simulink model "SlidesExampleNew"  (Simulink 7.4)
settings: Solver=FixedStepDiscrete  StartTime=0.0  StopTime=120  FixedStep=0.5  MaxStep=1  RelTol=1e-3
values from neighbouring files (symbols this model uses):
  y0 = -20    [SlidesExampleMfile.m]
undefined symbols (not defined in the file or in its folder): BLOM_FunctionCode, thetak, vk, xk, yk
libraries: BLOM_Lib x10
settings Model: Creator=vichik  LastModifiedBy=Kyle
settings OptimizationCC: InitFltsAndDblsToZero=on
settings DebuggingCC: StrictBusMsg=ErrorLevel1

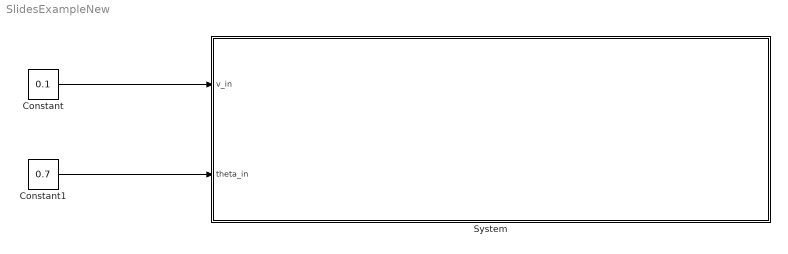
== system SlidesExampleNew ==
  Constant : Constant  Value=0.1
  Constant1 : Constant  Value=0.7
  System : Subsystem
  wires:
  Constant/1 -> System/1(v_in)
  Constant1/1 -> System/2(theta_in)

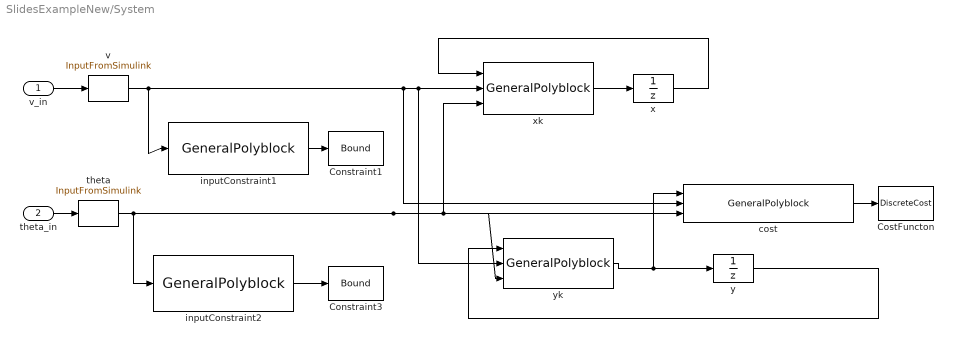
== system SlidesExampleNew/System ==
  v_in : Inport
  theta_in : Inport  Port=2
  Constraint1 : BLOM_Lib/Bound  SystemSampleTime=-1  ub=0  lb=-inf  initial_step=on  intermediate_step=on  final_step=on
  Constraint3 : BLOM_Lib/Bound  SystemSampleTime=-1  ub=0  lb=-inf  initial_step=on  intermediate_step=on  final_step=on
  CostFuncton : BLOM_Lib/DiscreteCost  SystemSampleTime=-1  initial_step=on  intermediate_step=on  final_step=on
  cost : BLOM_Lib/GeneralPolyblock  SystemSampleTime=-1  P_f=[0 2 0; 0 0 2;2 0 0;1 0 0;0 0 0]  K_f=[1 1 1 -10 25]  P_g=[0 0 0]  K_g=1  inputs=yk,vk,thetak  inputScalar=on  outputScalar=on
  inputConstraint1 : BLOM_Lib/GeneralPolyblock  SystemSampleTime=-1  P_f="[1  ;  0 ]"  K_f=[1 -1 ; -1 0]  P_g=[0 ]  K_g=1  inputs=v  inputScalar=on  outputScalar=off
  inputConstraint2 : BLOM_Lib/GeneralPolyblock  SystemSampleTime=-1  P_f=[1;0]  K_f="[1 -pi/2; -1  0]"  P_g=[0]  K_g=1  inputs=theta  inputScalar=on  outputScalar=off
  theta : BLOM_Lib/InputFromSimulink  SystemSampleTime=-1  interpType=Zero-Order Hold
  v : BLOM_Lib/InputFromSimulink  SystemSampleTime=-1  interpType=Zero-Order Hold
  x : UnitDelay  SampleTime=-1
  xk : BLOM_Lib/GeneralPolyblock  SystemSampleTime=-1  P_f=[1 0 0;0 1 BLOM_FunctionCode('cos')]  K_f=[1 0.5]  P_g=[0 0 0]  K_g=1  inputs=xk,vk,thetak  inputScalar=on  outputScalar=on
  y : UnitDelay  X0=y0  SampleTime=-1
  yk : BLOM_Lib/GeneralPolyblock  SystemSampleTime=-1  P_f=[1 0 0; 0 1 BLOM_FunctionCode('sin')]  K_f=[1 0.5]  P_g=[0 0 0]  K_g=1  inputs=yk,vk,thetak  inputScalar=on  outputScalar=on
  wires:
  xk/1 -> x/1
  x/1 -> xk/1
  v/1 -> cost/2, xk/2, yk/2, inputConstraint1/1
  cost/1 -> CostFuncton/1
  v_in/1 -> v/1
  inputConstraint1/1 -> Constraint1/1
  theta_in/1 -> theta/1
  theta/1 -> inputConstraint2/1, xk/3, cost/3, yk/3
  yk/1 -> cost/1, y/1
  y/1 -> yk/1
  inputConstraint2/1 -> Constraint3/1
